simulink model "shunt_active_filter"  (Simulink 7.5)
settings: Solver=ode1  StartTime=0.0  StopTime=0.2  RelTol=1e-3
libraries: powerlib x13, dsparch4 x1
settings Model: Creator=Jawad  LastModifiedBy=Arpit

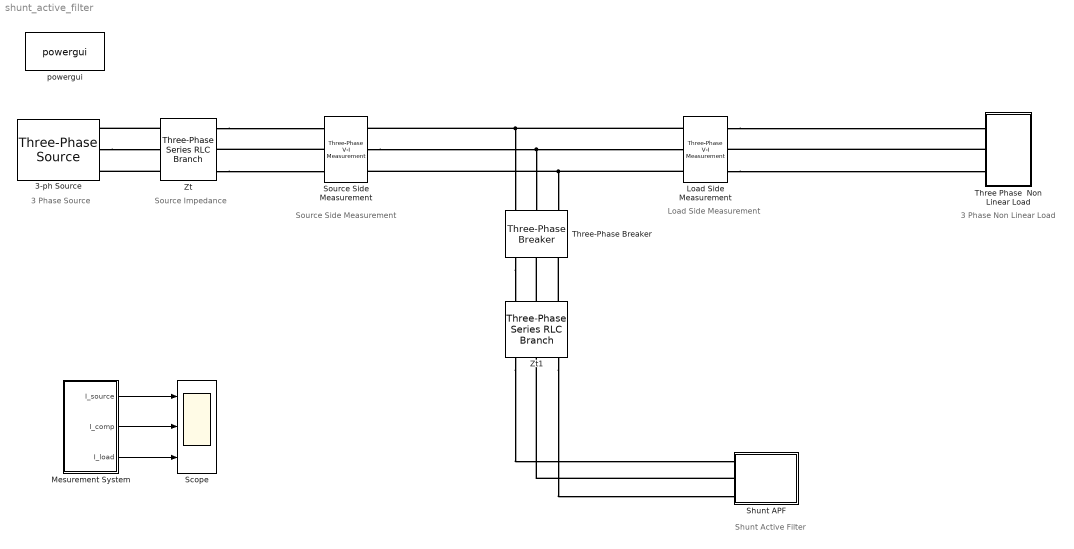
== system shunt_active_filter ==
  note: 3 Phase
      | Source
  note: 3 Phase
      | Non Linear Load
  note: Shunt Active Filter
  note: Load Side
      | Measurement
  note: Source Side
      | Measurement
  note: Source
      | Impedance
  3-ph Source : powerlib/Electrical Sources/Three-Phase Source  DialogController=POWERSYS.PowerSysDialog  SystemSampleTime=-1  Voltage=400  PhaseAngle=0  Frequency=50  InternalConnection=Yg  SpecifyImpedance=off  Resistance=0.001  Inductance=1e-8  ShortCircuitLevel=100e6  BaseVoltage=25e3  XRratio=7
  Load Side Measurement : powerlib/Measurements/Three-Phase V-I Measurement  DialogController=POWERSYS.PowerSysDialog  SystemSampleTime=-1  VoltageMeasurement=phase-to-ground  SetLabelV=on  LabelV=Vload  Vpu=off  VpuLL=off  CurrentMeasurement=yes  SetLabelI=on  LabelI=Iload  Ipu=off  Pbase=100e6  Vbase=500e3  OutputType=Complex  PhasorSimulation=off  PSBequivalent=0
      link override Model/VI/Ia: GotoTag=LibraryTag_Ia
      link override Model/VI/Ib: GotoTag=LibraryTag_Ib
      link override Model/VI/Ic: GotoTag=LibraryTag_Ic
      link override Model/VI/Va: GotoTag=LibraryTag_Va
      link override Model/VI/Vb: GotoTag=LibraryTag_Vb
      link override Model/VI/Vc: GotoTag=LibraryTag_Vc
  Mesurement System : Subsystem
  Scope : Scope  NumInputPorts=3
      settings: TickLabels=on  YMin=-70~-35~-75  YMax=70~35~75  SaveName=ScopeData3
  Shunt APF : Subsystem
  Source Side Measurement : powerlib/Measurements/Three-Phase V-I Measurement  DialogController=POWERSYS.PowerSysDialog  SystemSampleTime=-1  VoltageMeasurement=phase-to-ground  SetLabelV=on  LabelV=Vs  Vpu=off  VpuLL=off  CurrentMeasurement=yes  SetLabelI=on  LabelI=Is  Ipu=off  Pbase=100e6  Vbase=500e3  OutputType=Complex  PhasorSimulation=off  PSBequivalent=0
      link override Model/VI/Ia: GotoTag=LibraryTag_Ia
      link override Model/VI/Ib: GotoTag=LibraryTag_Ib
      link override Model/VI/Ic: GotoTag=LibraryTag_Ic
      link override Model/VI/Va: GotoTag=LibraryTag_Va
      link override Model/VI/Vb: GotoTag=LibraryTag_Vb
      link override Model/VI/Vc: GotoTag=LibraryTag_Vc
  Three Phase  Non Linear Load : Subsystem
  Three-Phase Breaker : powerlib/Elements/Three-Phase Breaker  DialogController=POWERSYS.PowerSysDialog  SystemSampleTime=-1  InitialState=open  SwitchA=on  SwitchB=on  SwitchC=on  SwitchTimes=0.04  External=off  BreakerResistance=1e-6  SnubberResistance=1e6  SnubberCapacitance=inf  Measurements=None
  Zt : powerlib/Elements/Three-Phase Series RLC Branch  DialogController=POWERSYS.PowerSysDialog  PhysicalDomain=powersysdomain  SubClassName=unknown  LeftPortType=p1  RightPortType=p1  LConnTagsString=A|B|C  RConnTagsString=A|B|C  BranchType=RL  Resistance=0.01  Inductance=1e-6  Capacitance=1e-6  Measurements=None
  Zt1 : powerlib/Elements/Three-Phase Series RLC Branch  DialogController=POWERSYS.PowerSysDialog  PhysicalDomain=powersysdomain  SubClassName=unknown  LeftPortType=p1  RightPortType=p1  LConnTagsString=A|B|C  RConnTagsString=A|B|C  BranchType=L  Resistance=0.01  Inductance=5e-3  Capacitance=1e-6  Measurements=None
  powergui : powerlib/powergui  Priority=1  SystemSampleTime=-1  SimulationMode=Discrete  SampleTime=5e-6  frequency=60  SPID=off  DisableSnubberDevices=off  DisableRonSwitches=off  DisableVfSwitches=off  SwTol=0  Interpol=off  frequencyindice=50  echomessages=off  HookPort=off  DisplayEquations=off  FunctionMessages=off  EnableUseOfTLC=off  x0status=blocks  RestoreLinks=warning  ResistiveCurrentMeasurement=off  Ylog=off  Xlog=on  ShowGrid=off  save=off  variable=ZData  structure=Load_Current  ZoomFFT=off  StartTime=0.06  cycles=4  DisplayStyle=2  fundamental=50  FreqAxis=off  MaxFrequency=1000  frequencyindicesteady=1  display=off  methode=off
  wires:
  Mesurement System/1(I_source) -> Scope/1
  Mesurement System/3(I_load) -> Scope/3
  Mesurement System/2(I_comp) -> Scope/2
  connections:
  Zt/RConn1 -- Source Side Measurement/LConn1
  Source Side Measurement/LConn2 -- Zt/RConn2
  Zt/RConn3 -- Source Side Measurement/LConn3
  Zt/LConn1 -- 3-ph Source/RConn1
  3-ph Source/RConn2 -- Zt/LConn2
  Zt/LConn3 -- 3-ph Source/RConn3
  Load Side Measurement/LConn1 -- Source Side Measurement/RConn1 -- Three-Phase Breaker/LConn1
  Load Side Measurement/LConn3 -- Source Side Measurement/RConn3 -- Three-Phase Breaker/LConn3
  Source Side Measurement/RConn2 -- Load Side Measurement/LConn2 -- Three-Phase Breaker/LConn2
  Three-Phase Breaker/RConn1 -- Zt1/RConn1
  Zt1/RConn2 -- Three-Phase Breaker/RConn2
  Zt1/RConn3 -- Three-Phase Breaker/RConn3
  Zt1/LConn1 -- Shunt APF/LConn1
  Shunt APF/LConn2 -- Zt1/LConn2
  Zt1/LConn3 -- Shunt APF/LConn3
  Load Side Measurement/RConn3 -- Three Phase  Non Linear Load/LConn3
  Three Phase  Non Linear Load/LConn2 -- Load Side Measurement/RConn2
  Load Side Measurement/RConn1 -- Three Phase  Non Linear Load/LConn1

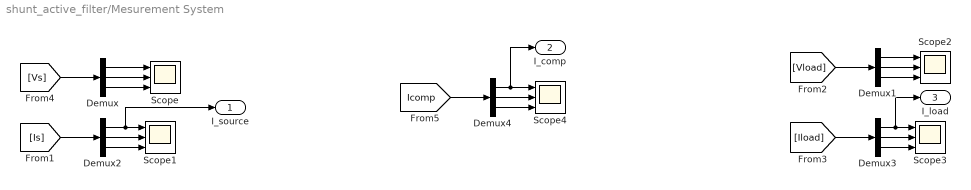
== system shunt_active_filter/Mesurement System ==
  Demux{,1..4} (5 alike) : Demux  Outputs=3
  Scope{,1..4} (5 alike) : Scope  NumInputPorts=3
      Scope settings: YMin=-5~-5~-5  YMax=5~5~5
      Scope1 settings: YMin=-5~-5~-5  YMax=5~5~5  SaveName=Source_Current
      Scope2 settings: YMin=-5~-5~-5  YMax=5~5~5  SaveName=ScopeData4
      Scope3 settings: YMin=-5~-5~-5  YMax=5~5~5  SaveName=Load_Current
      Scope4 settings: YMin=-5~-5~-5  YMax=5~5~5  SaveName=ScopeData6
  I_source : Outport
  I_comp : Outport  Port=2
  I_load : Outport  Port=3
  wires:
  [Vs] -> Demux/1
  [Is] -> Demux2/1
  [Vload] -> Demux1/1
  [Iload] -> Demux3/1
  Demux/3 -> Scope/3
  Demux/2 -> Scope/2
  Demux/1 -> Scope/1
  Demux2/1 -> Scope1/1, I_source/1
  Demux2/2 -> Scope1/2
  Demux2/3 -> Scope1/3
  Demux1/3 -> Scope2/3
  Demux1/2 -> Scope2/2
  Demux1/1 -> Scope2/1
  Demux3/1 -> Scope3/1, I_load/1
  Demux3/2 -> Scope3/2
  Demux3/3 -> Scope3/3
  [Icomp] -> Demux4/1
  Demux4/1 -> Scope4/1, I_comp/1
  Demux4/2 -> Scope4/2
  Demux4/3 -> Scope4/3

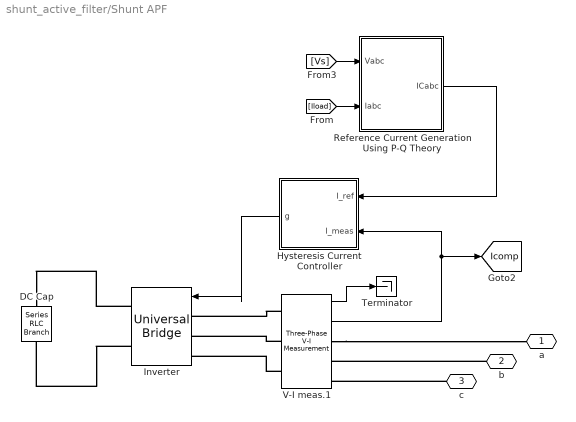
== system shunt_active_filter/Shunt APF ==
  DC Cap : powerlib/Elements/Series RLC Branch  DialogController=POWERSYS.PowerSysDialog  PhysicalDomain=powersysdomain  SubClassName=unknown  LeftPortType=p1  RightPortType=p1  LConnTagsString=__new0  RConnTagsString=__new0  BranchType=C  Resistance=1  Inductance=1e-3  SetiL0=off  InitialCurrent=0  Capacitance=40e-6  Setx0=off  InitialVoltage=400  Measurements=None
  Hysteresis Current Controller : Subsystem
  Inverter : powerlib/Power Electronics/Universal Bridge  DialogController=POWERSYS.PowerSysDialog  SystemSampleTime=-1  Arms=3  SnubberResistance=10000  SnubberCapacitance=inf  Device=IGBT / Diodes  Ron=1e-4  Lon=0  ForwardVoltages="[  1  1  ]"  ForwardVoltage=.8  GTOparameters=[ 10e-6 , 20e-6 ]  IGBTparameters=[ 1e-6 , 2e-6 ]  Measurements=None  Measurements_2=None  converterType=Rectifier
  Reference Current Generation Using P-Q Theory : Subsystem
  Terminator : Terminator
  V-I meas.1 : powerlib/Measurements/Three-Phase V-I Measurement  DialogController=POWERSYS.PowerSysDialog  SystemSampleTime=-1  VoltageMeasurement=phase-to-ground  SetLabelV=off  LabelV=Vabc  Vpu=off  VpuLL=off  CurrentMeasurement=yes  SetLabelI=off  LabelI=Iabc  Ipu=off  Pbase=100e6  Vbase=500e3  OutputType=Complex  PhasorSimulation=off  PSBequivalent=0
      link override Model/VI/Ia: GotoTag=LibraryTag_Ia
      link override Model/VI/Ib: GotoTag=LibraryTag_Ib
      link override Model/VI/Ic: GotoTag=LibraryTag_Ic
      link override Model/VI/Va: GotoTag=LibraryTag_Va
      link override Model/VI/Vb: GotoTag=LibraryTag_Vb
      link override Model/VI/Vc: GotoTag=LibraryTag_Vc
  a : PMIOPort  Port=1  Side=Left
  b : PMIOPort  Port=2  Side=Left
  c : PMIOPort  Port=3  Side=Left
  tag scope: Icomp=global
  wires:
  [Vs] -> Reference Current Generation Using P-Q Theory/1(Vabc)
  Hysteresis Current Controller/1(g) -> Inverter/1
  [Iload] -> Reference Current Generation Using P-Q Theory/2(Iabc)
  Reference Current Generation Using P-Q Theory/1(ICabc) -> Hysteresis Current Controller/1(I_ref)
  V-I meas.1/1 -> Terminator/1
  V-I meas.1/2 -> Hysteresis Current Controller/2(I_meas), [Icomp]
  connections:
  Inverter/RConn1 -- DC Cap/LConn1
  V-I meas.1/LConn1 -- Inverter/LConn1
  V-I meas.1/LConn2 -- Inverter/LConn2
  V-I meas.1/LConn3 -- Inverter/LConn3
  Inverter/RConn2 -- DC Cap/RConn1
  V-I meas.1/RConn1 -- a/RConn1
  b/RConn1 -- V-I meas.1/RConn2
  c/RConn1 -- V-I meas.1/RConn3

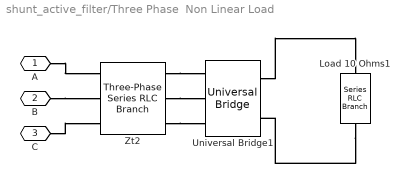
== system shunt_active_filter/Three Phase  Non Linear Load ==
  Load 10 Ohms1 : powerlib/Elements/Series RLC Branch  DialogController=POWERSYS.PowerSysDialog  PhysicalDomain=powersysdomain  SubClassName=unknown  LeftPortType=p1  RightPortType=p1  LConnTagsString=__new0  RConnTagsString=__new0  BranchType=R  Resistance=10  Inductance=0.1  SetiL0=off  InitialCurrent=0  Capacitance=[]  Setx0=off  InitialVoltage=0  Measurements=None
  Universal Bridge1 : powerlib/Power Electronics/Universal Bridge  DialogController=POWERSYS.PowerSysDialog  SystemSampleTime=-1  Arms=3  SnubberResistance=1e5  SnubberCapacitance=1e-10  Device=Diodes  Ron=1e-3  Lon=0  ForwardVoltages="[  0  0  ]"  ForwardVoltage=0  GTOparameters=[ 10e-6 , 20e-6 ]  IGBTparameters=[ 1e-6 , 2e-6 ]  Measurements=None  Measurements_2=None  converterType=Rectifier
  Zt2 : powerlib/Elements/Three-Phase Series RLC Branch  DialogController=POWERSYS.PowerSysDialog  PhysicalDomain=powersysdomain  SubClassName=unknown  LeftPortType=p1  RightPortType=p1  LConnTagsString=A|B|C  RConnTagsString=A|B|C  BranchType=RL  Resistance=0.01  Inductance=1e-4  Capacitance=1e-6  Measurements=None
  A : PMIOPort  Port=1  Side=Left
  B : PMIOPort  Port=2  Side=Left
  C : PMIOPort  Port=3  Side=Left
  connections:
  Universal Bridge1/RConn1 -- Load 10 Ohms1/LConn1
  Load 10 Ohms1/RConn1 -- Universal Bridge1/RConn2
  Zt2/RConn1 -- Universal Bridge1/LConn1
  Zt2/RConn2 -- Universal Bridge1/LConn2
  Zt2/RConn3 -- Universal Bridge1/LConn3
  A/RConn1 -- Zt2/LConn1
  B/RConn1 -- Zt2/LConn2
  C/RConn1 -- Zt2/LConn3

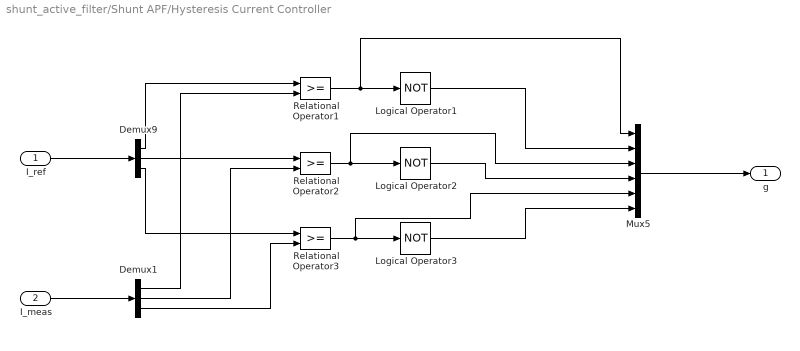
== system shunt_active_filter/Shunt APF/Hysteresis Current Controller ==
  I_ref : Inport
  I_meas : Inport  Port=2
  Demux1 : Demux  Outputs=3
  Demux9 : Demux  Outputs=3
  Logical Operator1 : Logic  Operator=NOT  AllPortsSameDT=off  OutDataTypeMode=boolean  OutDataTypeStr=boolean
  Logical Operator2 : Logic  Operator=NOT  AllPortsSameDT=off  OutDataTypeMode=boolean  OutDataTypeStr=boolean
  Logical Operator3 : Logic  Operator=NOT  AllPortsSameDT=off  OutDataTypeMode=boolean  OutDataTypeStr=boolean
  Mux5 : Mux  Inputs=6
  Relational Operator1 : RelationalOperator  LogicOutDataTypeMode=boolean  LogicDataType=fixdt(0, 8)  OutDataTypeStr=boolean
  Relational Operator2 : RelationalOperator  LogicOutDataTypeMode=boolean  LogicDataType=fixdt(0, 8)  OutDataTypeStr=boolean
  Relational Operator3 : RelationalOperator  LogicOutDataTypeMode=boolean  LogicDataType=fixdt(0, 8)  OutDataTypeStr=boolean
  g : Outport
  wires:
  Relational Operator1/1 -> Logical Operator1/1, Mux5/1
  Relational Operator2/1 -> Logical Operator2/1, Mux5/3
  Relational Operator3/1 -> Logical Operator3/1, Mux5/5
  Demux9/1 -> Relational Operator1/1
  Demux9/3 -> Relational Operator3/1
  Logical Operator1/1 -> Mux5/2
  Logical Operator2/1 -> Mux5/4
  Logical Operator3/1 -> Mux5/6
  Mux5/1 -> g/1
  Demux9/2 -> Relational Operator2/1
  Demux1/1 -> Relational Operator1/2
  Demux1/2 -> Relational Operator2/2
  Demux1/3 -> Relational Operator3/2
  I_ref/1 -> Demux9/1
  I_meas/1 -> Demux1/1

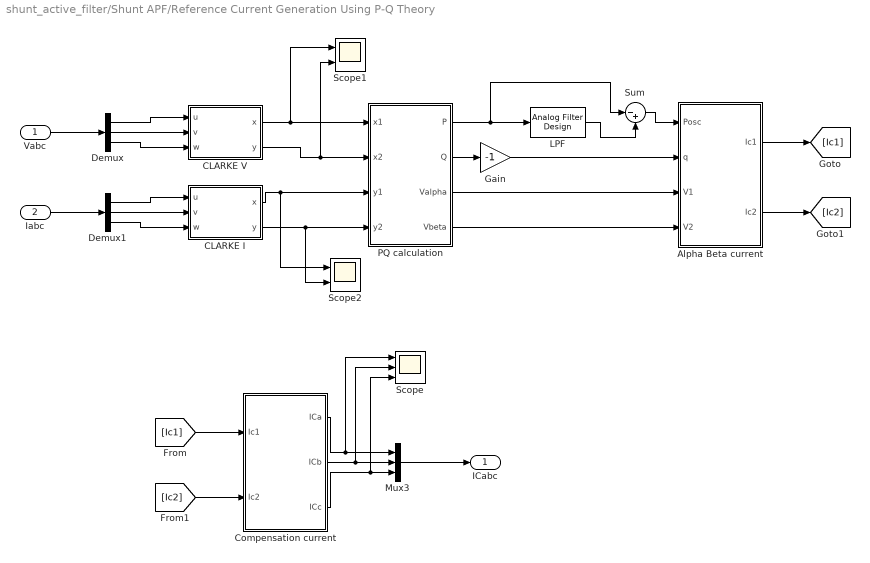
== system shunt_active_filter/Shunt APF/Reference Current Generation Using P-Q Theory ==
  Vabc : Inport
  Iabc : Inport  Port=2
  Alpha Beta current : Stateflow chart  TreatAsAtomicUnit=on
  CLARKE I : Stateflow chart  TreatAsAtomicUnit=on
  CLARKE V : Stateflow chart  TreatAsAtomicUnit=on
  Compensation current : Stateflow chart  TreatAsAtomicUnit=on
  Demux : Demux  Outputs=3
  Demux1 : Demux  Outputs=3
  Gain : Gain  Gain=-1  ParameterDataType=fixdt(1, 16)  ParameterScaling=2^0  OutDataType=fixdt(1, 16)  OutScaling=2^0
  LPF : dsparch4/Analog Filter Design  method=Butterworth  filttype=Lowpass  N=5  Wlo=2*pi*50  Whi=80  Rp=2  Rs=40
  Mux3 : Mux  Inputs=3
  PQ calculation : Stateflow chart  TreatAsAtomicUnit=on
  Scope : Scope  NumInputPorts=3
      settings: YMin=-35~-30~-30  YMax=30~35~35
  Scope1 : Scope  NumInputPorts=2
      settings: YMin=-400~-400  YMax=400~400  SaveName=ScopeData2
  Scope2 : Scope  NumInputPorts=2
      settings: TimeRange=0.2  YMin=-70~-80  YMax=70~80  SaveName=ScopeData5
  Sum : Sum  Inputs=|-+  OutDataType=fixdt(1, 16)  OutScaling=2^0
  ICabc : Outport
  wires:
  Iabc/1 -> Demux1/1
  Vabc/1 -> Demux/1
  [Ic1] -> Compensation current/1(Ic1)
  [Ic2] -> Compensation current/2(Ic2)
  Compensation current/1(ICa) -> Mux3/1, Scope/1
  Compensation current/2(ICb) -> Mux3/2, Scope/2
  Compensation current/3(ICc) -> Mux3/3, Scope/3
  CLARKE V/1(x) -> PQ calculation/1(x1), Scope1/1
  CLARKE V/2(y) -> PQ calculation/2(x2), Scope1/2
  CLARKE I/1(x) -> PQ calculation/3(y1), Scope2/1
  PQ calculation/2(Q) -> Gain/1
  PQ calculation/1(P) -> LPF/1, Sum/1
  Gain/1 -> Alpha Beta current/2(q)
  PQ calculation/3(Valpha) -> Alpha Beta current/3(V1)
  Alpha Beta current/1(Ic1) -> [Ic1]
  Alpha Beta current/2(Ic2) -> [Ic2]
  CLARKE I/2(y) -> PQ calculation/4(y2), Scope2/2
  PQ calculation/4(Vbeta) -> Alpha Beta current/4(V2)
  Demux/1 -> CLARKE V/1(u)
  Demux/2 -> CLARKE V/2(v)
  Demux/3 -> CLARKE V/3(w)
  Demux1/1 -> CLARKE I/1(u)
  Demux1/2 -> CLARKE I/2(v)
  Demux1/3 -> CLARKE I/3(w)
  Sum/1 -> Alpha Beta current/1(Posc)
  Mux3/1 -> ICabc/1
  LPF/1 -> Sum/2

== matlab function Shunt APF/Reference Current Generation Using P-Q Theory/CLARKE I ==
  data: u input double; x output double; v input double; w input double; y output double
function [x,y] = ICT(u,v,w)
%#em1

x = sqrt(2/3)*(u-(0.5*v)-(0.5*w));
y = sqrt(2)*(0+(0.5*v)-(0.5*w));

== matlab function Shunt APF/Reference Current Generation Using P-Q Theory/CLARKE V ==
  data: u input double; x output double; v input double; w input double; y output double
function [x,y] = VCT(u,v,w)
%#em1

x = sqrt(2/3)*(u-(0.5*v)-(0.5*w));
y = sqrt(2)*(0+(0.5*v)-(0.5*w));

== matlab function Shunt APF/Reference Current Generation Using P-Q Theory/PQ calculation ==
  data: x1 input double; P output double; Q output double; x2 input double; y1 input double; y2 input double; Valpha output double; Vbeta output double
function [P,Q,Valpha,Vbeta] = PQ(x1,x2,y1,y2)
%#em1

P = (x1*y1)+(x2*y2);
Q = (x2*y1)-(x1*y2);
Valpha = x1;
Vbeta = x2;

== matlab function Shunt APF/Reference Current Generation Using P-Q Theory/Compensation current ==
  data: Ic1 input double; ICa output double; Ic2 input double; ICb output double; ICc output double
function [ICa,ICb,ICc] = Ical(Ic1,Ic2)
%#em1

ICa = sqrt(2/3)*(Ic1);
ICb = sqrt(2/3)*((-0.5*Ic1)+((sqrt(3)/2)*Ic2));
ICc = sqrt(2/3)*((-0.5*Ic1)-((sqrt(3)/2)*Ic2));

== matlab function Shunt APF/Reference Current Generation Using P-Q Theory/Alpha Beta current ==
  data: Posc input double; Ic1 output double; q input double; V1 input double; Ic2 output double; V2 input double
function [Ic1,Ic2] = ICOM(Posc,q,V1,V2)
%#em1

Ic1 = (-1/(V1^2 + V2^2))*((Posc*V1)+(q*V2));
Ic2 = (-1/(V1^2 + V2^2))*((Posc*V2)-(q*V1));
